simulink model "orbit_simulink_v91"  (R2018a)
settings: Solver=ode5  StartTime=0.0  StopTime=51  FixedStep=0.0005  RelTol=1e-8  EnableMultiTasking=on
libraries: simulink x1
settings Model: ExtModeTrigMode=oneshot  ExtModeArmWhenConnect=off  Creator=lsi  LastModifiedBy=siguhe
settings DataIOCC: SaveFormat=Array  SignalLoggingSaveFormat=ModelDataLogs  SaveState=on
settings OptimizationCC: BlockReduction=off  BooleanDataType=off  ExpressionDepthLimit=2147483647  InitFltsAndDblsToZero=on  LifeSpan=inf
settings DebuggingCC: SaveWithParameterizedLinksMsg=none  UnderspecifiedInitializationDetection=Classic  MergeDetectMultiDrivingBlocksExec=none  SignalResolutionControl=TryResolveAllWithWarning  MultiTaskDSMMsg=warning  MultiTaskCondExecSysMsg=none  FcnCallInpInsideContextMsg=warning  StateNameClashWarn=warning  LibraryContextMissingDiagnostic=warning  SFUnexpectedBacktrackingDiag=warning  SFNoUnconditionalDefaultTransitionDiag=warning  SFExecutionAtInitializationDiag=none
settings HardwareCC: ProdBitPerPointer=32  ProdBitPerSizeT=32  ProdBitPerPtrDiffT=32  ProdLargestAtomicFloat=None  ProdIntDivRoundTo=Undefined  ProdEndianess=Unspecified  ProdWordSize=32  ProdHWDeviceType=32-bit Generic  TargetUnknown=on
settings ModelReferenceCC: PropagateSignalLabelsOutOfModel=off
settings CodeAppCC: StateflowObjectComments=on
settings GRTTargetCC: TargetLangStandard=C89/C90 (ANSI)  GeneratePreprocessorConditionals=Disable all  CombineOutputUpdateFcns=off  GRTInterface=on
settings ConfigComp: CovMetricSettings=dw  CovHtmlReporting=on  CovSaveCumulativeToWorkspaceVar=on  CovSaveSingleToWorkspaceVar=on  CovExternalEMLEnable=off

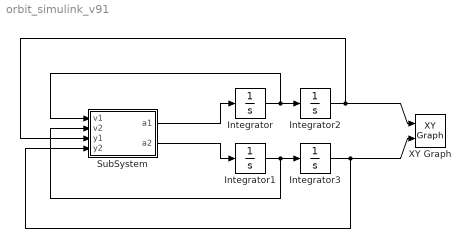
== system orbit_simulink_v91 ==
  Integrator : Integrator
  Integrator1 : Integrator  InitialCondition=-2.00158510637908252240537862224
  Integrator2 : Integrator  InitialCondition=0.994
  Integrator3 : Integrator
  SubSystem : Subsystem
  XY Graph : simulink/Sinks/XY Graph  xmin=-2  xmax=2  ymin=-2  ymax=2  st=-1
  wires:
  Integrator3/1 -> SubSystem/4(y2), XY Graph/2
  Integrator2/1 -> SubSystem/3(y1), XY Graph/1
  Integrator/1 -> Integrator2/1, SubSystem/1(v1)
  Integrator1/1 -> Integrator3/1, SubSystem/2(v2)
  SubSystem/1(a1) -> Integrator/1
  SubSystem/2(a2) -> Integrator1/1

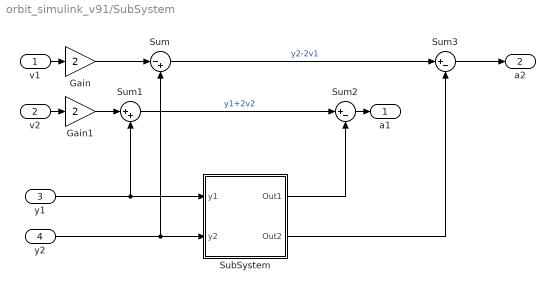
== system orbit_simulink_v91/SubSystem ==
  v1 : Inport
  v2 : Inport  Port=2
  y1 : Inport  Port=3
  y2 : Inport  Port=4
  Gain : Gain  Gain=2  SaturateOnIntegerOverflow=on  OutDataTypeStr=Inherit: Same as input  ParamDataTypeStr=Inherit: Same as input
  Gain1 : Gain  Gain=2  SaturateOnIntegerOverflow=on  OutDataTypeStr=Inherit: Same as input  ParamDataTypeStr=Inherit: Same as input
  SubSystem : Subsystem
  Sum : Sum  Inputs=|-+  SaturateOnIntegerOverflow=on  InputSameDT=on  OutDataTypeStr=Inherit: Same as first input
  Sum1 : Sum  Inputs=|++  SaturateOnIntegerOverflow=on  InputSameDT=on  OutDataTypeStr=Inherit: Same as first input
  Sum2 : Sum  Inputs=|+-  SaturateOnIntegerOverflow=on  InputSameDT=on  OutDataTypeStr=Inherit: Same as first input
  Sum3 : Sum  Inputs=|+-  SaturateOnIntegerOverflow=on  InputSameDT=on  OutDataTypeStr=Inherit: Same as first input
  a1 : Outport
  a2 : Outport  Port=2
  wires:
  v2/1 -> Gain1/1
  v1/1 -> Gain/1
  Gain/1 -> Sum/1
  y2/1 -> SubSystem/2(y2), Sum/2
  y1/1 -> SubSystem/1(y1), Sum1/2
  Gain1/1 -> Sum1/1
  Sum1/1 -> Sum2/1  "y1+2v2"
  Sum2/1 -> a1/1
  SubSystem/1(Out1) -> Sum2/2
  Sum/1 -> Sum3/1  "y2-2v1"
  SubSystem/2(Out2) -> Sum3/2
  Sum3/1 -> a2/1

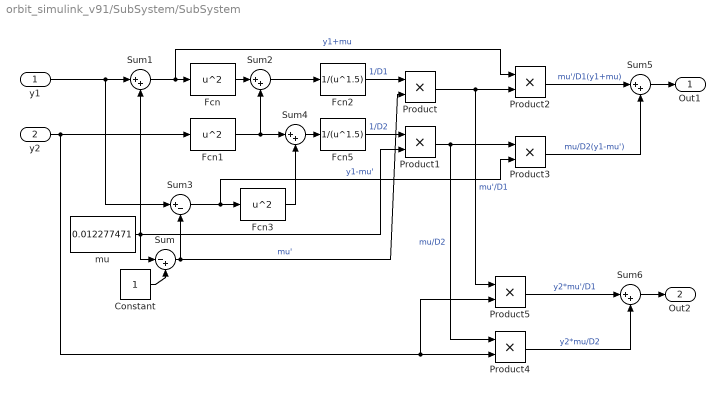
== system orbit_simulink_v91/SubSystem/SubSystem ==
  y1 : Inport
  y2 : Inport  Port=2
  Constant : Constant
  Fcn : Fcn  Expr=u^2
  Fcn1 : Fcn  Expr=u^2
  Fcn2 : Fcn  Expr=1/(u^1.5)
  Fcn3 : Fcn  Expr=u^2
  Fcn5 : Fcn  Expr=1/(u^1.5)
  Product{,1..5} (6 alike) : Product  SaturateOnIntegerOverflow=on  RndMeth=Zero  InputSameDT=on  OutDataTypeStr=Inherit: Same as first input
  Sum : Sum  Inputs=|-+  SaturateOnIntegerOverflow=on  InputSameDT=on  OutDataTypeStr=Inherit: Same as first input
  Sum{1..2,4..6} (5 alike) : Sum  Inputs=|++  SaturateOnIntegerOverflow=on  InputSameDT=on  OutDataTypeStr=Inherit: Same as first input
  Sum3 : Sum  Inputs=|+-  SaturateOnIntegerOverflow=on  InputSameDT=on  OutDataTypeStr=Inherit: Same as first input
  mu : Constant  Value=0.012277471
  Out1 : Outport
  Out2 : Outport  Port=2
  wires:
  Constant/1 -> Sum/2
  Sum2/1 -> Fcn2/1
  Fcn/1 -> Sum2/1
  Fcn1/1 -> Sum2/2, Sum4/1
  Sum4/1 -> Fcn5/1
  Fcn5/1 -> Product1/1  "1/D2"
  Fcn2/1 -> Product/1  "1/D1"
  Sum1/1 -> Fcn/1, Product2/1  "y1+mu"
  Fcn3/1 -> Sum4/2
  Sum3/1 -> Fcn3/1, Product3/2  "y1-mu'"
  Product2/1 -> Sum5/1  "mu'/D1(y1+mu)"
  Product3/1 -> Sum5/2  "mu/D2(y1-mu')"
  y2/1 -> Fcn1/1, Product4/2, Product5/2
  Product5/1 -> Sum6/1  "y2*mu'/D1"
  Product4/1 -> Sum6/2  "y2*mu/D2"
  y1/1 -> Sum1/1, Sum3/1
  mu/1 -> Sum1/2, Product1/2, Sum/1
  Product1/1 -> Product3/1, Product4/1  "mu/D2"
  Product/1 -> Product2/2, Product5/1  "mu'/D1"
  Sum5/1 -> Out1/1
  Sum6/1 -> Out2/1
  Sum/1 -> Sum3/2, Product/2  "mu'"
